simulink model "test_transmission"  (R2015a)
settings: Solver=ode3  SolverMode=SingleTasking  StartTime=0.0  StopTime=10.0  RelTol=1e-3
settings Model: ExtModeTrigDuration=2  Creator=kkhoo  LastModifiedBy=kkhoo
settings OptimizationCC: OptimizeModelRefInitCode=on  LifeSpan=1
settings DebuggingCC: UnderspecifiedInitializationDetection=Classic  MergeDetectMultiDrivingBlocksExec=none
settings HardwareCC: ProdBitPerInt=16  ProdBitPerPointer=8  ProdIntDivRoundTo=Zero  ProdEndianess=LittleEndian  ProdWordSize=8  ProdHWDeviceType=Atmel->AVR
settings RTWCC: SystemTargetFile=realtime.tlc  GenerateMakefile=off  TemplateMakefile=realtime.tmf  Description=Run on Target Hardware  RTWVerbose=off  CustomSource=src/Engduino.h src/engduino_wrappers.cpp
settings ERTTargetCC: CombineOutputUpdateFcns=off  ExtModeTransport=3  ExtModeMexFile=ext_serial_win32_comm_rtt  ExtModeMexArgs=0 1 9600  ERTSrcFileBannerTemplate=realtime_code_template.cgt  ERTHdrFileBannerTemplate=realtime_code_template.cgt  ERTDataSrcFileTemplate=realtime_code_template.cgt  ERTDataHdrFileTemplate=realtime_code_template.cgt  ERTCustomFileTemplate=realtime_file_process.tlc

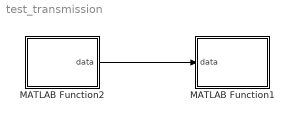
== system test_transmission ==
  MATLAB Function1 : MATLAB Function  LoadFcn=|  TreatAsAtomicUnit=on  mask(Button){}
      | set_param(gcs, 'CustomSource', strjoin(unique([strsplit(get_param(gcs, 'CustomSource')) ...
      |  'src/engduino_wrappers.cpp' 'src/Engduino.h'])));
      mask help: Outputs 1 if the button is pressed, 0 otherwise.
  MATLAB Function2 : MATLAB Function  LoadFcn=|  TreatAsAtomicUnit=on  mask(Button){}
      | set_param(gcs, 'CustomSource', strjoin(unique([strsplit(get_param(gcs, 'CustomSource')) ...
      |  'src/engduino_wrappers.cpp' 'src/Engduino.h'])));
      mask help: Outputs 1 if the button is pressed, 0 otherwise.
  wires:
  MATLAB Function2/1(data) -> MATLAB Function1/1(data)

== matlab function test_transmission/MATLAB Function1 ==
  data: data input
function print_serial(data)

if strcmp(coder.target, 'rtw')
    coder.ceval('print_data_serial_wrapper', data);
end

== matlab function test_transmission/MATLAB Function2 ==
  data: data output
function data = read_serial()

data = 0;

if strcmp(coder.target, 'rtw')
    data = coder.ceval('read_data_serial_wrapper');
end
